simulink model "soac_autocode_test"  (R2018b)
settings: Solver=VariableStepAuto  StartTime=0.0  StopTime=10.0  RelTol=1e-3
undefined symbols (not defined in the file): exitcode, s, soar_count, soar_interface_lib, soar_params, time, U, X
libraries: simulink x2, dspswit3 x1, soar_lib x1
settings Model: Creator=taylorreynolds  LastModifiedBy=taylorreynolds
settings OptimizationCC: DefaultParameterBehavior=Inlined  UseDivisionForNetSlopeComputation=on  UseFloatMulNetSlope=on  InlineInvariantSignals=on  PassReuseOutputArgsAs=Individual arguments  ZeroExternalMemoryAtStartup=off  ZeroInternalMemoryAtStartup=off  NoFixptDivByZeroProtection=on  EfficientFloat2IntCast=on  LifeSpan=1
settings DebuggingCC: ParameterTunabilityLossMsg=error
settings HardwareCC: ProdBitPerPointer=32  ProdBitPerSizeT=32  ProdBitPerPtrDiffT=32  ProdLargestAtomicInteger=Long  ProdLargestAtomicFloat=Double  ProdWordSize=32  ProdLongLongMode=on  ProdHWDeviceType=NXP->Cortex-M4
settings SFSimCC: SimUseLocalCustomCode=off  MATLABDynamicMemAlloc=off
settings RTWCC: SystemTargetFile=ert.tlc  TemplateMakefile=ert_default_tmf  GenerateReport=on  RTWUseLocalCustomCode=off  CustomInclude=/Users/taylorreynolds/SOCI/soci-gnc/Lib/FSW/adcs_oac/include/ecos/include  BuildConfiguration=Faster Runs  IncludeHyperlinkInReport=on  LaunchReport=on  GenerateTraceInfo=on  GenerateTraceReport=on  GenerateTraceReportSl=on  GenerateTraceReportSf=on  GenerateTraceReportEml=on  GenerateCodeMetricsReport=on
settings RTWCC: CustomSource=|
  | /Users/taylorreynolds/SOCI/soci-gnc/Lib/FSW/adcs_oac/include/ecos/src/amd_1.c
  | /Users/taylorreynolds/SOCI/soci-gnc/Lib/FSW/adcs_oac/include/ecos/src/amd_2.c
  | /Users/taylorreynolds/SOCI/soci-gnc/Lib/FSW/adcs_oac/include/ecos/src/amd_aat.c
  | /Users/taylorreynolds/SOCI/soci-gnc/Lib/FSW/adcs_oac/include/ecos/src/amd_control.c
  | /Users/taylorreynolds/SOCI/soci-gnc/Lib/FSW/adcs_oac/include/ecos/src/amd_defaults.c
  | /Users/taylorreynolds/SOCI/soci-gnc/Lib/FSW/adcs_oac/include/ecos/src/amd_dump.c
  | /Users/taylorreynolds/SOCI/soci-gnc/Lib/FSW/adcs_oac/include/ecos/src/amd_global.c
  | /Users/taylorreynolds/SOCI/soci-gnc/Lib/FSW/adcs_oac/include/ecos/src/amd_info.c
  | /Users/taylorreynolds/SOCI/soci-gnc/Lib/FSW/adcs_oac/include/ecos/src/amd_order.c
  | /Users/taylorreynolds/SOCI/soci-gnc/Lib/FSW/adcs_oac/include/ecos/src/amd_post_tree.c
  | /Users/taylorreynolds/SOCI/soci-gnc/Lib/FSW/adcs_oac/include/ecos/src/amd_postorder.c
  | /Users/taylorreynolds/SOCI/soci-gnc/Lib/FSW/adcs_oac/include/ecos/src/amd_preprocess.c
  | /Users/taylorreynolds/SOCI/soci-gnc/Lib/FSW/adcs_oac/include/ecos/src/amd_valid.c
  | /Users/taylorreynolds/SOCI/soci-gnc/Lib/FSW/adcs_oac/include/ecos/src/cone.c
  | /Users/taylorreynolds/SOCI/soci-gnc/Lib/FSW/adcs_oac/include/ecos/src/ctrlc.c
  | /Users/taylorreynolds/SOCI/soci-gnc/Lib/FSW/adcs_oac/include/ecos/src/ecos.c
  | /Users/taylorreynolds/SOCI/soci-gnc/Lib/FSW/adcs_oac/include/ecos/src/equil.c
  | /Users/taylorreynolds/SOCI/soci-gnc/Lib/FSW/adcs_oac/include/ecos/src/expcone.c
  | /Users/taylorreynolds/SOCI/soci-gnc/Lib/FSW/adcs_oac/include/ecos/src/kkt.c
  | /Users/taylorreynolds/SOCI/soci-gnc/Lib/FSW/adcs_oac/include/ecos/src/ldl.c
  | /Users/taylorreynolds/SOCI/soci-gnc/Lib/FSW/adcs_oac/include/ecos/src/matlab_main.c
  | /Users/taylorreynolds/SOCI/soci-gnc/Lib/FSW/adcs_oac/include/ecos/src/preproc.c
  | /Users/taylorreynolds/SOCI/soci-gnc/Lib/FSW/adcs_oac/include/ecos/src/runecos.c
  | /Users/taylorreynolds/SOCI/soci-gnc/Lib/FSW/adcs_oac/include/ecos/src/spla.c
  | /Users/taylorreynolds/SOCI/soci-gnc/Lib/FSW/adcs_oac/include/ecos/src/splamm.c
  | /Users/taylorreynolds/SOCI/soci-gnc/Lib/FSW/adcs_oac/include/ecos/src/wright_omega.c
settings CodeAppCC: ForceParamTrailComments=on  IgnoreCustomStorageClasses=off  OperatorAnnotations=on  SimulinkDataObjDesc=on  SFDataObjDesc=on  CustomSymbolStrGlobalVar=rt$N$M  CustomSymbolStrType=$N$M  CustomSymbolStrFcn=$N$M$F  CustomSymbolStrMacro=$N$M  InsertBlockDesc=on
settings ERTTargetCC: TargetLangStandard=C99 (ISO)  MultiwordLength=2048  GenerateSampleERTMain=on  IncludeMdlTerminateFcn=off  CombineSignalStateStructs=on  SupportAbsoluteTime=off  SupportComplex=off  SupportNonInlinedSFcns=on  InlinedParameterPlacement=NonHierarchical  ERTCustomFileTemplate=example_file_process.tlc  ERTFilePackagingFormat=CompactWithDataFile

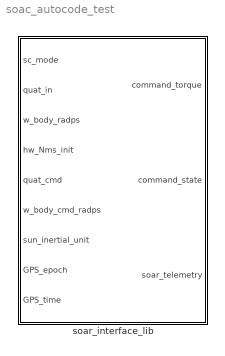
== system soac_autocode_test ==
  soar_interface_lib : Subsystem  AncestorBlock=soar_interface_lib/soar_interface_lib

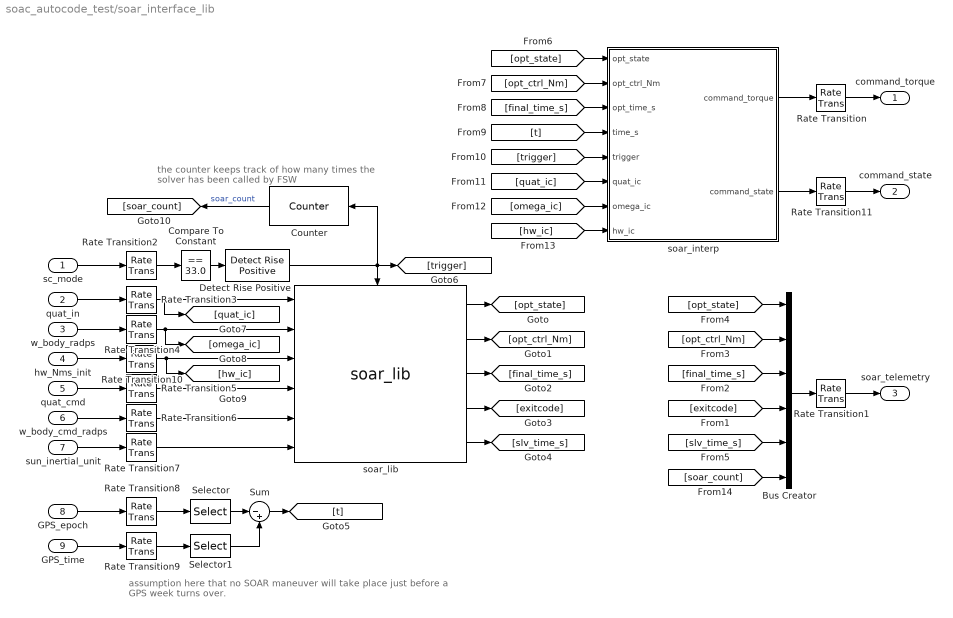
== system soac_autocode_test/soar_interface_lib ==
  note: the counter keeps track of how many times
      | the solver has been called by FSW
  note: assumption here that no SOAR maneuver will take place just
      | before a GPS week turns over.
  sc_mode : Inport
  quat_in : Inport  Port=2
  w_body_radps : Inport  Port=3
  hw_Nms_init : Inport  Port=4
  quat_cmd : Inport  Port=5
  w_body_cmd_radps : Inport  Port=6
  sun_inertial_unit : Inport  Port=7
  GPS_epoch : Inport  Port=8
  GPS_time : Inport  Port=9
  Bus Creator : BusCreator  Inputs=X,U,s,exitcode,time,soar_count
  Compare To Constant : simulink/Logic and Bit Operations/Compare To Constant  relop===  const=33.0  OutDataTypeStr=boolean
  Counter : dspswit3/Counter  Direction=Up  CountEvent=Rising edge  CounterSize=32 bits  MaxCount=255  InitialCount=0  Output=Count  HitValue=32  ResetInput=off  SamplesPerFrame=1  Ts=1  CntDtype=uint32  HitDtype=Logical
  Detect Rise Positive : simulink/Logic and Bit Operations/Detect Rise Positive  vinit=0  OutDataTypeStr=boolean
  Rate Transition : RateTransition  InitialCondition=soar_params.ic.cmd_torque
  Rate Transition1 : RateTransition
  Rate Transition10 : RateTransition  InitialCondition=soar_params.ic.hw_Nms  OutPortSampleTime=soar_params.sample_time_s
  Rate Transition11 : RateTransition  InitialCondition=soar_params.ic.cmd_state
  Rate Transition2 : RateTransition  InitialCondition=soar_params.ic.sc_mode  OutPortSampleTime=soar_params.sample_time_s
  Rate Transition3 : RateTransition  InitialCondition=soar_params.ic.quat_in  OutPortSampleTime=soar_params.sample_time_s
  Rate Transition4 : RateTransition  InitialCondition=soar_params.ic.w_body_radps  OutPortSampleTime=soar_params.sample_time_s
  Rate Transition5 : RateTransition  InitialCondition=soar_params.ic.quat_cmd  OutPortSampleTime=soar_params.sample_time_s
  Rate Transition6 : RateTransition  InitialCondition=soar_params.ic.w_body_cmd_radps  OutPortSampleTime=soar_params.sample_time_s
  Rate Transition7 : RateTransition  InitialCondition=soar_params.ic.sun_inertial_unit  OutPortSampleTime=soar_params.sample_time_s
  Rate Transition8 : RateTransition  InitialCondition=soar_params.ic.gps_epoch_s  OutPortSampleTime=soar_params.sample_time_s
  Rate Transition9 : RateTransition  InitialCondition=soar_params.ic.gps_time_s  OutPortSampleTime=soar_params.sample_time_s
  Selector : Selector  InputPortWidth=2  IndexOptions=Index vector (dialog)  Indices=1  OutputSizes=1
  Selector1 : Selector  InputPortWidth=2  IndexOptions=Index vector (dialog)  Indices=1  OutputSizes=1
  Sum : Sum  Inputs=|-+
  soar_interp : Subsystem
  soar_lib : soar_lib/soar_lib  SystemSampleTime=-1
  command_torque : Outport
  command_state : Outport  Port=2
  soar_telemetry : Outport  Port=3
  wires:
  soar_lib/3 -> [final_time_s]
  soar_lib/2 -> [opt_ctrl_Nm]
  hw_Nms_init/1 -> Rate Transition10/1
  Rate Transition10/1 -> [hw_ic], soar_lib/3
  Selector1/1 -> Sum/2
  Selector/1 -> Sum/1
  Rate Transition9/1 -> Selector1/1
  Rate Transition8/1 -> Selector/1
  Rate Transition7/1 -> soar_lib/6
  Rate Transition6/1 -> soar_lib/5
  Rate Transition5/1 -> soar_lib/4
  Rate Transition4/1 -> [omega_ic], soar_lib/2
  Rate Transition3/1 -> soar_lib/1, [quat_ic]
  Rate Transition1/1 -> soar_telemetry/1
  [opt_state] -> Bus Creator/1
  [opt_ctrl_Nm] -> Bus Creator/2
  [final_time_s] -> Bus Creator/3
  [exitcode] -> Bus Creator/4
  [slv_time_s] -> Bus Creator/5
  Bus Creator/1 -> Rate Transition1/1
  Sum/1 -> [t]
  GPS_time/1 -> Rate Transition9/1
  GPS_epoch/1 -> Rate Transition8/1
  soar_lib/4 -> [exitcode]
  soar_lib/5 -> [slv_time_s]
  soar_lib/1 -> [opt_state]
  Compare To Constant/1 -> Detect Rise Positive/1
  sc_mode/1 -> Rate Transition2/1
  sun_inertial_unit/1 -> Rate Transition7/1
  w_body_cmd_radps/1 -> Rate Transition6/1
  quat_cmd/1 -> Rate Transition5/1
  w_body_radps/1 -> Rate Transition4/1
  quat_in/1 -> Rate Transition3/1
  Rate Transition2/1 -> Compare To Constant/1
  soar_interp/1(command_torque) -> Rate Transition/1
  soar_interp/2(command_state) -> Rate Transition11/1
  Counter/1 -> [soar_count]  "soar_count"
  [opt_state] -> soar_interp/1(opt_state)
  [opt_ctrl_Nm] -> soar_interp/2(opt_ctrl_Nm)
  [final_time_s] -> soar_interp/3(opt_time_s)
  [t] -> soar_interp/4(time_s)
  [trigger] -> soar_interp/5(trigger)
  [quat_ic] -> soar_interp/6(quat_ic)
  [omega_ic] -> soar_interp/7(omega_ic)
  [hw_ic] -> soar_interp/8(hw_ic)
  Rate Transition/1 -> command_torque/1
  Rate Transition11/1 -> command_state/1
  Detect Rise Positive/1 -> Counter/1, [trigger], soar_lib/Trigger
  [soar_count] -> Bus Creator/6

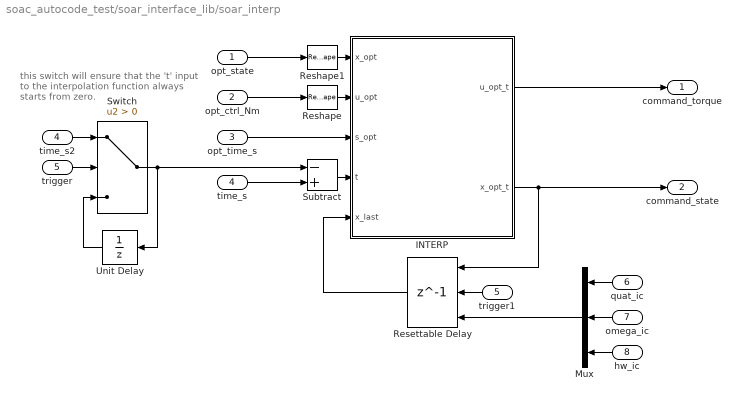
== system soac_autocode_test/soar_interface_lib/soar_interp ==
  note: this switch will ensure that the 't'
      | input to the interpolation function
      | always starts from zero.
  opt_state : Inport
  opt_ctrl_Nm : Inport  Port=2
  opt_time_s : Inport  Port=3
  time_s : Inport  Port=4
  trigger : Inport  Port=5
  quat_ic : Inport  Port=6
  omega_ic : Inport  Port=7
  hw_ic : Inport  Port=8
  INTERP : MATLAB Function  TreatAsAtomicUnit=on
  Mux : Mux  Inputs=[4 3 3]
  Resettable Delay : Delay  DelayLength=1  InitialConditionSource=Input port  ExternalReset=Rising
      settings: InputPortMap=u0,r5,p4
  Reshape : Reshape  OutputDimensionality=Customize  OutputDimensions=[3,soar_params.N]
  Reshape1 : Reshape  OutputDimensionality=Customize  OutputDimensions=[10,soar_params.N]
  Subtract : Sum  Inputs=-+
  Switch : Switch  Criteria=u2 > Threshold
  Unit Delay : UnitDelay  SampleTime=-1
  time_s2 : InportShadow  Port=4
  trigger1 : InportShadow  Port=5
  command_torque : Outport
  command_state : Outport  Port=2
  wires:
  time_s/1 -> Subtract/2
  quat_ic/1 -> Mux/1
  trigger1/1 -> Resettable Delay/2
  hw_ic/1 -> Mux/3
  Reshape/1 -> INTERP/2(u_opt)
  Switch/1 -> Unit Delay/1, Subtract/1
  Reshape1/1 -> INTERP/1(x_opt)
  opt_ctrl_Nm/1 -> Reshape/1
  Unit Delay/1 -> Switch/3
  time_s2/1 -> Switch/1
  omega_ic/1 -> Mux/2
  opt_state/1 -> Reshape1/1
  trigger/1 -> Switch/2
  opt_time_s/1 -> INTERP/3(s_opt)
  INTERP/2(x_opt_t) -> command_state/1, Resettable Delay/1
  Resettable Delay/1 -> INTERP/5(x_last)
  Subtract/1 -> INTERP/4(t)
  INTERP/1(u_opt_t) -> command_torque/1
  Mux/1 -> Resettable Delay/3

== matlab function soac_autocode_test/soar_interface_lib/soar_interp/INTERP ==
  data: u_opt_t output size=3; x_opt input; x_opt_t output size=10; u_opt input; s_opt input size=1; t input size=1; x_last input size=10; soar_params parameter
function [u_opt_t,x_opt_t] = soac_INTERP(x_opt,u_opt,s_opt,t,x_last,soar_params)
%SOAR_INTERP
%
% This function will interpolate the optimal solution from SOAR given the
% time t. Time t is assumed to represent the time SINCE the optimizer was
% called by flight software (necessitating the switch outside of this
% function). One RK4 step is performed to interpolate the state, while the
% control is interpolated using affine interpolation.
%
% T. Reynolds -- RAIN LAB

%#codegen

% parameters
N  = soar_params.N;
ut = linspace(0,s_opt,N);
k  = sum(t>ut); % current time interval
J  = soar_params.inertia; % kg m2

% Output final state and ZERO feedforward control if we are beyond the 
% final maneuver time
if ((s_opt>eps)&&(t>=s_opt))
    u_opt_t = zeros(3,1);
    x_opt_t = [ x_opt(1:4,N); J\x_opt(5:7,N); x_opt(8:10,N) ];
    return;
end

% Otherwise integrate to current state and interpolate for current control
if ((k>0) && (s_opt>eps))
    um      = u_opt(3*(k-1)+(1:3));
    up      = u_opt(3*k+(1:3));
    u       = [reshape(um,3,1) reshape(up,3,1)];
    tspan   = [ ut(k); ut(k+1) ];
    
    % step integrator for feedforward state x_opt_t
    x_opt_t = rk4_one_step(t,x_last,u,J,tspan,soar_params.sample_time_s);

    % interpolate for feedforward control u_opt_t
    u_opt_t = zeros(3,1);
    for i = 1:3
        u_opt_t(i) = interp1(ut,u_opt(i,:),t,'linear');
    end
else
    % this case happens when the optimizer has not yet been called
    u_opt_t = zeros(3,1);
    x_opt_t = x_last;
end

end % soar_interp

%%%%%%%%%%%%%%%%%%%%%%%%%%%%%%%%%%%%%%%%%%%%%%%%%%%%%%%%%%%%%%%%%%%%%%%%%%%
%%%%%%%%%%%%%%%%%%%%%%%%%%%% SUPPORT FUNCTIONS %%%%%%%%%%%%%%%%%%%%%%%%%%%%
%%%%%%%%%%%%%%%%%%%%%%%%%%%%%%%%%%%%%%%%%%%%%%%%%%%%%%%%%%%%%%%%%%%%%%%%%%%

function x = rk4_one_step(t,x,u,J,tspan,dt)
    
k1 = deriv(t     ,x        ,u,J,tspan);
k2 = deriv(t+dt/2,x+dt/2*k1,u,J,tspan);
k3 = deriv(t+dt/2,x+dt/2*k2,u,J,tspan);
k4 = deriv(t+dt  ,x+dt*k3  ,u,J,tspan);

x = (x+dt/6*(k1+2*k2+2*k3+k4));

end

function dx = deriv(t,x,u,J,tspan)

% States
q   = x(1:4)./norm(x(1:4));
q0  = q(1);
qv  = q(2:4);
w   = x(5:7);
hw  = x(8:10);

% interpolate u_opt at time t
tkm     = tspan(1);
tkp     = tspan(2);
lam_km  = (tkp - t)/(tkp - tkm);
lam_kp  = (t - tkm)/(tkp - tkm);
u_t     = lam_km .* u(:,1) + lam_kp .* u(:,2);

% Kinematics & Dynamics
fq  = 0.5 * [ -qv'; skew(qv)+q0*eye(3) ] * w;
fw  = J\(-u_t - skew(w) * (J*w + hw));
fhw = u_t;

dx = [ fq; fw; fhw ];

end
